simulink model "Load_Current_Limits"  (R2021b)
settings: Solver=FixedStepDiscrete  StartTime=0.0  StopTime=10  RelTol=1e-3
model workspace (MAT data in the model file):
  TsModel = 0.1
undefined symbols (not defined in the file): Curr_Test_Load, Voltage_Test_Vector
libraries: simulink x1
settings Model: ExtModeTrigDuration=8  Creator=vivekr  LastModifiedBy=vlenzi
settings SolverCC: AlgebraicLoopSolver=TrustRegion
settings DataIOCC: SaveFormat=StructureWithTime  SaveOutput=off  SignalLogging=off  DSMLogging=off  SaveTime=off  SignalLoggingName=logsOut
settings OptimizationCC: DefaultParameterBehavior=Inlined  UseDivisionForNetSlopeComputation=UseDivisionForReciprocalsOfIntegersOnly  EnhancedBackFolding=on  BooleansAsBitfields=on  PassReuseOutputArgsAs=Individual arguments  ExpressionDepthLimit=2147483647  StateBitsets=on  DataBitsets=on  ZeroExternalMemoryAtStartup=off  NoFixptDivByZeroProtection=on  EfficientFloat2IntCast=on  LifeSpan=1  MaxStackSize=64  SimCompilerOptimization=on  EfficientTunableParamExpr=on
settings DebuggingCC: ReadBeforeWriteMsg=DisableAll  WriteAfterWriteMsg=DisableAll  WriteAfterReadMsg=DisableAll  CheckExecutionContextPreStartOutputMsg=on  ParameterPrecisionLossMsg=none  UniqueDataStoreMsg=error  AllowSymbolicDim=off  ModelReferenceSymbolNameMessage=none  StateNameClashWarn=warning  StrictBusMsg=ErrorOnBusTreatedAsVector  SymbolicDimsDataTypeCodeGenerationDiagnostic=none  SFUnexpectedBacktrackingDiag=warning  SFNoUnconditionalDefaultTransitionDiag=warning  SFExecutionAtInitializationDiag=none  SFMachineParentedDataDiag=warning  ArithmeticOperatorsInVariantConditions=warning
settings HardwareCC: TargetHWDeviceType=Generic->32-bit Embedded Processor
settings ModelReferenceCC: CheckModelReferenceTargetMessage=none  PropagateSignalLabelsOutOfModel=off
settings SFSimCC: SimUseLocalCustomCode=off  MATLABDynamicMemAlloc=off
settings RTWCC: Description=Embedded Coder  SystemTargetFile=ert.tlc  TemplateMakefile=ert_default_tmf  GenerateReport=on  RTWVerbose=off  RTWUseLocalCustomCode=off  IncludeHyperlinkInReport=on  PortableWordSizes=on  CodeExecutionProfiling=on  CodeProfilingSaveOptions=AllData  CodeProfilingInstrumentation=coarse  GenerateTraceInfo=on  GenerateTraceReport=on  GenerateTraceReportSl=on  GenerateTraceReportSf=on  GenerateTraceReportEml=on  GenerateCodeMetricsReport=on
settings CodeAppCC: ForceParamTrailComments=on  IgnoreCustomStorageClasses=off  SimulinkDataObjDesc=on  CustomSymbolStrGlobalVar=rt$N$M  CustomSymbolStrType=$N$M  CustomSymbolStrFcn=$N$M$F  CustomSymbolStrMacro=$N$M  InsertBlockDesc=on  StateflowObjectComments=on  InternalIdentifier=Classic
settings ERTTargetCC: UtilityFuncGeneration=Shared location  MultiwordLength=2048  IncludeMdlTerminateFcn=off  CombineSignalStateStructs=on  SupportNonFinite=off  SupportComplex=off  ExtModeStaticAllocSize=2048  ERTCustomFileTemplate=example_file_process.tlc  ERTFilePackagingFormat=CompactWithDataFile  ConvertIfToSwitch=off  SuppressUnreachableDefaultCases=off
settings ConfigComp: CovMetricSettings=dw  CovSaveCumulativeToWorkspaceVar=on  CovSaveSingleToWorkspaceVar=on  CovExternalEMLEnable=off  CovSFcnEnable=off

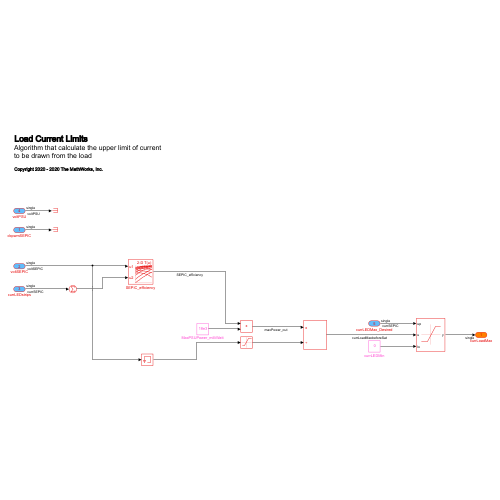
[thumbnail: Simulink's stored preview of the top-level diagram]
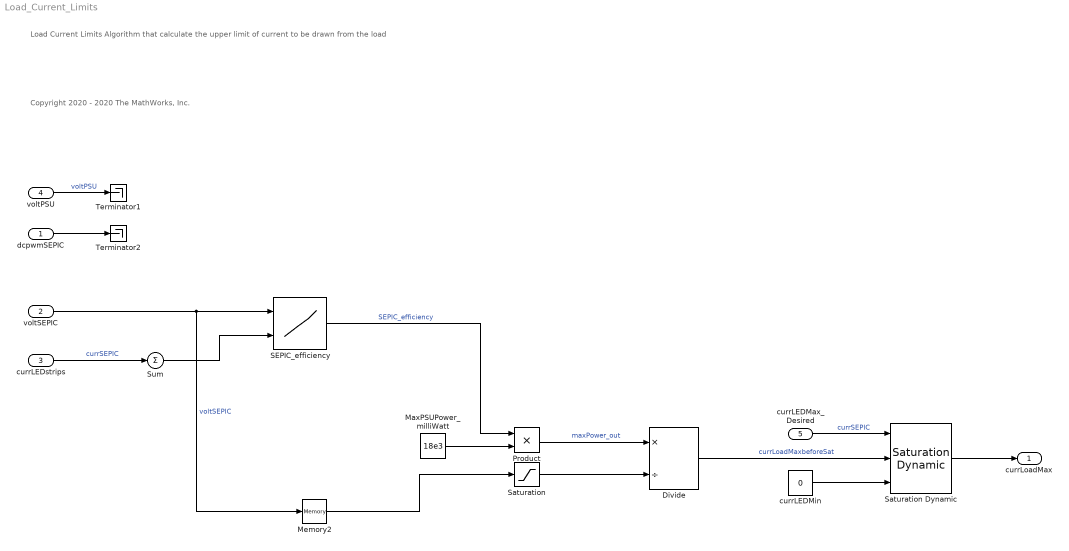
== system Load_Current_Limits ==
  note: Load Current Limits
      | Algorithm that calculate the upper limit of current to be drawn from the load
  note: Copyright 2020 - 2020 The MathWorks, Inc.
  dcpwmSEPIC : Inport  OutDataTypeStr=single  Unit=1  PortDimensions=1  SampleTime=TsModel
  voltSEPIC : Inport  Port=2  OutDataTypeStr=single  Unit=V  PortDimensions=1  SampleTime=TsModel
  currLEDstrips : Inport  Port=3  OutDataTypeStr=single  Unit=mA  PortDimensions=6  SampleTime=TsModel
  voltPSU : Inport  Port=4  OutDataTypeStr=single  Unit=V  PortDimensions=1  SampleTime=TsModel
  currLEDMax_Desired : Inport  Port=5  OutDataTypeStr=single  Unit=mA  PortDimensions=1  SampleTime=TsModel
  Divide : Product  Inputs=*/
  MaxPSUPower_milliWatt : Constant  Value=18e3  OutDataTypeStr=single
  Memory2 : Memory
  Product : Product
  SEPIC_efficiency : Lookup_n-D  BreakpointsForDimension1=Voltage_Test_Vector  BreakpointsForDimension2=Curr_Test_Load  Table=effMatrix'  ExtrapMethod=Clip  UseLastTableValue=on  InternalRulePriority=Speed  RndMeth=Simplest  InputSameDT=on
      settings: InputPortMap=u0,u1
  Saturation : Saturate  UpperLimit=50  LowerLimit=1e-3
  Saturation Dynamic : simulink/Discontinuities/Saturation Dynamic  OutMin=[]  OutMax=[]  OutDataTypeStr=Inherit: Same as second input  OutDataType=fixdt(1, 16)  OutScaling=2^-10  DoSatur=off
  Sum : Sum  Inputs=+
  Terminator1 : Terminator
  Terminator2 : Terminator
  currLEDMin : Constant  Value=0  OutDataTypeStr=single
  currLoadMax : Outport  OutDataTypeStr=single  Unit=mA  PortDimensions=1  SampleTime=TsModel
  wires:
  voltPSU/1 -> Terminator1/1  "voltPSU"
  voltSEPIC/1 -> Memory2/1, SEPIC_efficiency/1  "voltSEPIC"
  MaxPSUPower_milliWatt/1 -> Product/2
  Saturation/1 -> Divide/2
  dcpwmSEPIC/1 -> Terminator2/1
  currLEDstrips/1 -> Sum/1  "currSEPIC"
  Memory2/1 -> Saturation/1
  Divide/1 -> Saturation Dynamic/2  "currLoadMaxbeforeSat"
  SEPIC_efficiency/1 -> Product/1  "SEPIC_efficiency"
  Saturation Dynamic/1 -> currLoadMax/1
  currLEDMax_Desired/1 -> Saturation Dynamic/1  "currSEPIC"
  currLEDMin/1 -> Saturation Dynamic/3
  Sum/1 -> SEPIC_efficiency/2
  Product/1 -> Divide/1  "maxPower_out"
